simulink model "Boat_sim"  (Simulink 7.5)
settings: Solver=FixedStepDiscrete  StartTime=0.0  StopTime=1000  FixedStep=.01  RelTol=1e-3
InitFcn:
  | boat_constants
values from neighbouring files (symbols this model uses):
  C_d_sea_surge = 340    [boat_constants.m]
  d_prop = .4572    (= 0.4572)    [boat_constants.m]
  figure8_waypoints = int32([ ... (first row only)    [boat_constants.m]
  InitialPoint = 0    [boat_constants.m]    (also in l2plus.m)
  IPStar = 0    [boat_constants.m]    (also in l2plus.m)
  ISA_g = 9.815    [boat_constants.m]
  K_t = 0.5    [boat_constants.m]
  mass = 550    [boat_constants.m]
  MaxDwnPthStar = 1    [boat_constants.m]    (also in l2plus.m)
  OC2max = 49999    [boat_constants.m]    (also in simulation_constants.m)
  phi_0 = 0    [boat_constants.m]    (also in simulation_constants.m)
  rho_w = 1.03e3    (= 1030)    [boat_constants.m]
  sampling_waypoints = int32([ ... (first row only)    [boat_constants.m]
  switchDistance = 4    [boat_constants.m]    (also in l2plus.m)
  T_step = 0.01    [boat_constants.m]    (also in common.m)
  tanIntercept = tan( 45*pi/180 )    [boat_constants.m]    (also in l2plus.m)
  test_waypoints = int32([ ... (first row only)    [boat_constants.m]
  TStar = single(4.5)    [boat_constants.m]    (also in l2plus.m = single(2))
  Turn2Track = 0    [boat_constants.m]    (also in l2plus.m)
  wheelbase = 3.27    [boat_constants.m]
undefined symbols (not defined in the file or in its folder): clock, DiscIntNeverNeededParam, Earth, serial, WGS84
libraries: simulink x25, uSimLib x4, instrumentlib x3, aerolibconvert2 x2, aerolibtransform2 x1, aerolibanimutils x1, simulink_need_slupdate x1
(part 3 of 3)

== matlab function HIL Interface/Parse HIL input/Embedded MATLAB Function ==
  data: successCount output double; failCount output double; in input uint8; out output uint8 size=22
function [successCount, failCount, out] = parseMessage(in)
    persistent actuatorMessage internalSuccessCount internalFailCount;
    
    if isempty(actuatorMessage)
        actuatorMessage = zeros(22, 1, 'uint8');
        internalSuccessCount = uint32(0);
        internalFailCount = uint32(0);
    end
    
    for i = 1:size(in,1)
        [new fail data] = buildAndCheckMessage(in(i));
        if new
            actuatorMessage = data;
            internalSuccessCount = internalSuccessCount + 1;
        elseif fail
            internalFailCount = internalFailCount + 1;
        end
    end
    successCount = internalSuccessCount;
    failCount = internalFailCount;
    out = actuatorMessage;
end

function [new fail data] = buildAndCheckMessage(characterIn)
%#eml

    persistent message messageIndex messageState actuatorData;

    if isempty(message)
        message = zeros(29, 1, 'uint8');
        messageIndex = uint8(0);
        messageState = uint8(0);
        actuatorData = zeros(22, 1, 'uint8');
    end

    % This contains the function's state of whether
    % it is currently building a message.
    % 0 - Awaiting header byte 0 (%)
    % 1 - Awaiting header byte 1 (&)
    % 2 - Building message
    % 3 - Awaiting header byte 0 (^)
    % 4 - Awaiting header byte 1 (&)
    % 5 - Reading checksum character

    new = false;
    fail = false;

    % We start recording a new message if we see the header
    if messageState == 0
        if characterIn == '%'
            message(1) = characterIn;
            messageIndex = uint8(2);
            messageState = uint8(1);
        else
            fail = true;
        end
    elseif messageState == 1
        % If we don't find the necessary ampersand we start over
        % waiting for a new sentence
        if characterIn == '&'
            message(2) = characterIn;
            messageIndex = messageIndex + 1;
            messageState = uint8(2);
        elseif characterIn ~= '%'
            messageIndex = uint8(1);
            messageState = uint8(0);
            fail = true;
        end
    elseif messageState == 2
        % Record every character that comes in now that we're building a sentence.
        % Only stop if we run out of room or an asterisk is found.
        message(messageIndex) = characterIn;
        messageIndex = messageIndex + 1;
        if messageIndex > 4 && message(4) < 249 && messageIndex == message(4) + 6
            if characterIn == '^'
                messageState = uint8(3);
            else
                messageState = uint8(0);
                messageIndex = uint8(1);
                fail = true;
            end
        elseif messageIndex == length(message) - 1
            % If we've filled up the buffer, ignore the entire message as we can't store it all
            messageIndex = uint8(1);
            messageState = uint8(0);
            fail = true;
        end
    elseif messageState == 3
        % If we don't find the necessary ampersand we continue
        % recording data as we haven't found the footer yet until
        % we've filled up the entire message (ends at 124 characters
        % as we need room for the 2 footer chars).
        message(messageIndex) = characterIn;
        messageIndex = messageIndex + 1;
        if characterIn == '&'
            messageState = uint8(4);
        elseif messageIndex == length(message)
            messageState = uint8(0);
            messageIndex = uint8(1);
            fail = true;
        end
    elseif messageState == 4
        % Record the checksum byte.
        message(messageIndex) = characterIn;

        % The checksum is now verified and if successful the message
        % is stored in the appropriate struct.
        checksumCalculated = uint8(0);
        for i=3:messageIndex-3
            checksumCalculated = bitxor(checksumCalculated, message(i));
        end

        if message(messageIndex) == checksumCalculated
            % If we've found an actuator message, update our local data store
            if message(3) == 2
                actuatorData = message(5:26);
                new = true;
            end
        else
            fail = true;
        end

        % We clear all state variables here regardless of success.
        messageIndex = uint8(1);
        messageState = uint8(0);
        message = zeros(29,1,'uint8');
    end

    data = actuatorData;
end

== matlab function Subsystem/Autonomous Controller/Rudder Command/L2 Plus ref WP1 ==
  data: reset input double; L2Vec output single; waypoints input int16; mode input uint8; Puav input single size=3; Vxyz input single size=3; switchDistance parameter double size=1; ISA_g parameter double; tanIntercept parameter double; MaxDwnPthStar parameter double; Turn2Track parameter double; InitialPoint parameter double; IPStar parameter double; TStar parameter double; as_c output single; i0 output double; i1 output double; WP0 output double; WP1 output double
function [L2Vec, as_c, i0, i1, WP0, WP1] = L2PlusWP1(reset, waypoints, mode, Puav, Vxyz, switchDistance, ...
    ISA_g, tanIntercept, MaxDwnPthStar,Turn2Track,...
    InitialPoint, IPStar, TStar)
%==============================
%     computes bank angle command for following a straight line
%     by creating an aim point that may be more than L2 away 
%     from the UAV. The aim point is (usually) farther along the path 
%     toward WP1 than the UAV, and the intercept
%     angle is less than or equal to a specified value. This limits the intercept
%     angle even when the UAV is within L2 of the path.
%     See L2PlusWP1.m for details
    
%         INPUTS   
%             T1      unit vector WP0-->WP1
%             N1      normal to T1
%             WP0     position of "from" waypoint. only needed to set an InitialPoint
%             WP1     position of WP1, active waypoint
%             Puav    position of UAV
%             Vxyz    Inertial velocity
%             switchDistance distance from WP1 to switch to WP2

%         PARAMETERS
%             ISA_g   gravity
%             tanIntercept  tangent of intercept angle
%             MaxDwnPthStar L2 multiplier to determmine downpath aimpoint
%             Turn2Track    true to turn toward T1 instead of L2
%             InitialPoint  true if no line tracking at first--fly direct to some initial point
%             IPStar        L2 multiplier to determing distance of IP from first WP0
%             Tstar         was called L2Base, time constant of response
%             
%         OUTPUTS
%             phi_c   commanded bank angle (positive is a starboard turn)
%             L2Vec   L2 vector toward aim point
%             as_c    commanded lateral acceleration
%             Groundspeed 
%             IP1     position of IP for plotting purposes. IP1(3) = -999 if no IP exists

    persistent IPActive;  %true if flying toward IP
    persistent IP; % location of initial point

    persistent index_0 index_1; % Store the indices for waypoints 0 & 1 respectively
    persistent direction; % Keep track of the direction for patrol mode
    
    % Make sure we have at least two waypoints
    assert(size(waypoints,1) >= 2);

    % Inititalize to the first waypoint
    if isempty(index_0)
        index_0 = int8(1);
    end
    if isempty(index_1)
        index_1 = int8(2);
    end
    if isempty(direction)
        direction = int8(1);
    end
    
    % Reset the waypoints
    if (reset)
        index_0 = int8(1);
        index_1 = int8(2);
    end
    
    % Select the two current waypoints we're dealing with
    WP0 = single(waypoints(index_0,:)');
    WP1 = single(waypoints(index_1,:)');
    i0 = index_0;
    i1 = index_1;
    
    switchToNextWaypoint = false;
    Pwp1 = single(zeros(3,1));
    Pe_y = single(0);
    Dist2WP1 = single(0);
    MinDownPath = single(0);
    Dist2WPSwitch = single(0);
    L2DownPath = single(0);
    L2ToT = single(zeros(3,1));
    L2Vec = single(zeros(3,1));
    IP1 = single([0; 0;-999]); %signal for no IP
    
    Pne = [Puav(1); Puav(2); 0]; %horizontal position
    Vne = [Vxyz(1); Vxyz(2); 0]; % horizontal velocity
    Groundspeed = norm(Vne);
    L2 = single(TStar*Groundspeed);
    WP0ne = single(zeros(3,1));
    
% Calculate N1 and T1
assert(norm(WP1 - WP0) ~= 0);
T1 = WP1-WP0;
T1 = T1/norm(T1);
N1 = [-T1(2); T1(1); 0];
    
%     initialize IP
    if (isempty(IPActive))
        if (InitialPoint)
%             IP is set relative to the first "from" waypoint
            IPActive = -1;
            IP = [WP0(1); WP0(2); 0] - L2*IPStar*T1;
            
            if (norm(IP-Pne) < .001)
                IPActive = 0;
                IP = single([0; 0; -999]);
            end
        else
            IPActive = 0;
            IP = single([0; 0;-999]); %signal for no IP
        end
    end
    IP1 = IP;
    
    
    if (IPActive)
%         no line tracking, direct to IP
        L2Vec = L2*(IP - Pne)/norm(IP - Pne);
%         check to see if at the IP to terminate this mode
        if norm(IP - Pne) < .1*L2
            IPActive = 0;
        end
    else
         if (Pne(1) < 2)
             IP1 = IP1;
         end
%         IP not active, track WP lines
        WPOne = [WP1(1); WP1(2); 0];
        Pwp1 = Pne - [WP1(1); WP1(2); 0]; % position of UAV relative to WP1
        Pe_y = single(Pwp1'*N1); % cross track error
        Dist2WP1 = -single(Pwp1'*T1); % distance to WP1

%         minimum down path distance for Aim Point intersection on T
%         is determined by the intercept angle but limited 
%         in case of very distant intecepts to MaxDwnPthStar*L2
        MinDownPath = single ( min( abs(Pe_y)/tanIntercept, MaxDwnPthStar*L2)); 
        Dist2WPSwitch = Dist2WP1 - switchDistance;
        if ( abs(Pe_y) > L2 )
    %             Make sure aimpoint is no closer to waypoint than calculated switch point.
            L2DownPath = MinDownPath;
        else
    %             within L2 of T and Dist2WPSwitch >= 0, but limit angle of L2 wrt T
            L2DownPath = (max(MinDownPath, (sqrt( L2^2 - Pe_y^2 ))));
        end
        
        if ( Dist2WPSwitch < 0 )
            switchToNextWaypoint = true;
        end
        
         % vector from Pwp1 to aim point on T1
         L2ToT = single(( Dist2WP1 - L2DownPath )*(-T1) - Pwp1);
         if (norm(L2ToT) < .001)
             L2Vec = L2*T1;
         else
            L2Vec = single(L2*( L2ToT/norm(L2ToT) )); % limit size to L2
         end
    %         L2Vec = L2ToT;
%         dummy statements
    end
    Zprod = single(Vxyz(1)*L2Vec(2) - Vxyz(2)*L2Vec(1)); %Z component of cross product
    sinEta = single(Zprod/(Groundspeed*L2));

    as_c = single(2*Groundspeed^2/(L2)*sinEta);
%         bank angle limits outside of this block
    phi_c = single(atan(as_c/ISA_g));

%         now override bank angle if heading in the wrong direction
    if ( Turn2Track && Dist2WPSwitch > 0 && ~IPActive ) 
%             turn to track not L2, gives min displacement from track
        if ( T1'*Vxyz < 0 )
            if ( Pe_y > 0 )
                phi_c = single(+pi/2);
                as_c = single(99);
            else
                phi_c = single(-pi/2);
                as_c = single(-99);
            end
        end
     else
%           turn toward L2, give min displacement toward WP0
        if ( L2Vec'*Vxyz < 0 )
            if ( sinEta < 0 )
                phi_c = single(-pi/2); 
                as_c = single(-99);
            else
                phi_c = single(+pi/2);
                as_c = single(99);
            end
        end
    end

% Now we process waypoint switching. This relies on the switchTrigger
% value set in the above L2+ controller code.
theEnd = false;
if index_1 + 1 <= size(waypoints,1) && waypoints(index_1+1,1) == -1 ...
                                    && waypoints(index_1+1,2) == -1 ...
                                    && waypoints(index_1+1,3) == -1
    theEnd = true;
end
if switchToNextWaypoint
    switch mode
        case 0 % Halt mode
            if size(waypoints,1) >= index_1 + 1 && ~theEnd
                index_0 = index_1;
                index_1 = index_1 + 1;
            end
        case 1 % Loop mode
            % We either continue moving forward through the waypoints...
            if size(waypoints,1) >= index_1 + 1 && ~theEnd
                index_0 = index_1;
                index_1 = index_1 + 1;
            % Or we wrap-around to the starting waypoint
            else
                index_0 = index_1;
                index_1 = int8(1);
            end
        case 2 % Patrol mode
            if direction == 1 % For the forwards direction
                % We either continue moving forwards through the waypoints...
                if size(waypoints,1) >= index_1 + 1 && ~theEnd
                    index_0 = index_1;
                    index_1 = index_1 + 1;
                % Or we start to go backwards
                else
                    index_0 = index_1;
                    index_1 = index_1 - 1;
                    direction = int8(0);
                end
            elseif direction == 0 % For the reverse direction
                % We either continue moving backwards through the waypoints...
                if index_1 - 1 >= 1
                    index_0 = index_1;
                    index_1 = index_1 - 1;
                % Or we start to go forwards
                else
                    index_0 = index_1;
                    index_1 = index_1 + 1;
                    direction = int8(1);
                end
            end
    end
end

== matlab function Subsystem/Select current waypoint track ==
  data: reset output double; nextTrack input double; resetTrackNumber input double; test_waypoints parameter double; figure8_waypoints parameter double; sampling_waypoints parameter double; waypoints output double
function [reset, waypoints] = selectTrack(nextTrack, resetTrackNumber, test_waypoints, figure8_waypoints, sampling_waypoints)
%#eml


% Initialize trackNumber.
% This variable is our state, which is the set of waypoints we're navigating
% between.
persistent trackNumber;
if isempty(trackNumber)
    trackNumber = uint8(1);
end

% Here is the logic for switching tracks. trackReset resets the trackNumber
% and nextTrack increments the track number
if resetTrackNumber
    trackNumber = uint8(1);
    reset = true;
elseif nextTrack
    trackNumber = trackNumber + uint8(1);
    if trackNumber > 3
        trackNumber = uint8(1);
    end
    reset = true;
else
    reset = false;
end

% 1 is for the test waypoints, 2 is for the figure eight, and 3 is
% for the data gathering waypoints.
switch trackNumber
    case 1
        waypoints = test_waypoints;
    case 2
        waypoints = figure8_waypoints;
    case 3
        waypoints = sampling_waypoints;
    otherwise
        waypoints = zeros(size(test_waypoints), 'int32');
end

== matlab function HIL Interface/Parse HIL input/Unpack sensor data ==
  data: u input uint8; rudderEnable output double; rudderDirection output double; rudderUp output double; rudderPeriod output double; ballastEnable output double; ballastDirection output double; throttleIdentifier output double; throttleData output double; throttleSize output double; throttleTrigger output double; timestamp output double
function [rudderEnable, rudderDirection, rudderUp, rudderPeriod, ballastEnable, ballastDirection, throttleIdentifier, throttleData, throttleSize, throttleTrigger, timestamp] = unpack(u)
%#eml

rudderEnable = u(1);
rudderDirection = u(2);
rudderUp = typecast(u(3:4), 'uint16');
rudderPeriod = typecast(u(5:6), 'uint16');
ballastEnable = u(7);
ballastDirection = u(8);
throttleIdentifier = typecast(u(9:12), 'uint32');
throttleData = u(13:18);
throttleSize = u(19);
throttleTrigger = u(20);
timestamp = typecast(u(21:22), 'uint16');

== matlab function HIL Interface/Pack ==
  data: speed input double; lat input double; lon input double; alt input double; yr input double; mon input double; day input double; hr input double; min input double; sec input double; cog input double; sog input double; newData input double; y output double; rudderPosition input double; rudderStarboardLimit input double; rudderPortLimit input double; ballastPosition input double; ballastStarboardLimit input double; ballastPortLimit input double; timestamp input double
function y = u(speed, lat, lon, alt, yr, mon, day, hr, min, sec, cog, sog, newData, rudderPosition, rudderStarboardLimit, rudderPortLimit, ballastPosition, ballastStarboardLimit, ballastPortLimit, timestamp)
%#eml

y = zeros(39, 1, 'uint8');
y(1:2) = typecast(speed, 'uint8');
y(3:6) = typecast(lat, 'uint8');
y(7:10) = typecast(lon, 'uint8');
y(11:14) = typecast(alt, 'uint8');
y(15) = yr;
y(16) = mon;
y(17) = day;
y(18) = hr;
y(19) = min;
y(20) = sec;
y(21:24) = typecast(cog, 'uint8');
y(25:28) = typecast(sog, 'uint8');
y(29) = newData;
y(30:31) = typecast(rudderPosition, 'uint8');
y(32) = rudderStarboardLimit;
y(33) = rudderPortLimit;
y(34:35) = typecast(ballastPosition, 'uint8');
y(36) = ballastStarboardLimit;
y(37) = ballastPortLimit;
y(38:39) = typecast(timestamp, 'uint8');

== matlab function Subsystem/Autonomous Controller/Rudder Command/Embedded MATLAB Function ==
  data: u input double; y output double
function y = fcn(u)
%#eml

y = atan2(u(2), u(1)) * 180 / pi;

== matlab function Subsystem/Log state data to workspace/Build HIL sentence/Pack ==
  data: a input double; y output double; b input double; c input double; d input double; e input double; f input double; g input double
function y = fcn(a, b, c, d, e, f, g)
%#eml

y = uint8([a;b;c;d;e;f;g]);

== matlab function Subsystem/Log state data to workspace/Pack ==
  data: L2 input double; y output double; gPos input double; head input double; lPos input double; vel input double
function y = fcn(L2, gPos, head, lPos, vel)
%#eml

y = zeros(52, 1, 'uint8');
y(1:4) = packUint32BE(typecast(L2(1),'uint32'));
y(5:8) = packUint32BE(typecast(L2(2),'uint32'));
y(9:12) = packUint32BE(typecast(L2(3),'uint32'));
y(13:16) = packUint32BE(typecast(gPos(1),'uint32'));
y(17:20) = packUint32BE(typecast(gPos(2),'uint32'));
y(21:24) = packUint32BE(typecast(gPos(3),'uint32'));
y(25:28) = packUint32BE(typecast(head,'uint32'));
y(29:32) = packUint32BE(typecast(lPos(1),'uint32'));
y(33:36) = packUint32BE(typecast(lPos(2),'uint32'));
y(37:40) = packUint32BE(typecast(lPos(3),'uint32'));
y(41:44) = packUint32BE(typecast(vel(1),'uint32'));
y(45:48) = packUint32BE(typecast(vel(2),'uint32'));
y(49:52) = packUint32BE(typecast(vel(3),'uint32'));

function out = packUint32BE(in)
out = zeros(4, 1, 'uint8');
out(1) = uint8(bitand(bitshift(in,-24),hex2dec('FF')));
out(2) = uint8(bitand(bitshift(in,-16),hex2dec('FF')));
out(3) = uint8(bitand(bitshift(in,-8),hex2dec('FF')));
out(4) = uint8(bitand(in,hex2dec('FF')));

== matlab function HIL Interface/Parse HIL input/Embedded MATLAB Function2 ==
  data: u1 input double; y output double; u2 input double
function y = safeDiv(u1, u2)
%#eml

if u2 == 0
    y = u1;
else
    y = u1 / u2;
end

== matlab function Subsystem/Autonomous Controller/Throttle Command/Mux Everything/Select data packet ==
  data: y output double; dis input double; en input double
function y = fcn(dis, en)
% This block controls the switch selecting between enable, 
% disable, and speed commands. If disable and enable are
% both set high, disable overrides anything else.

y = uint8(3);
if dis == 1
    y = uint8(1);
elseif en == 1
    y = uint8(2);
end
